simulink model "PAlab3_2_6"  (R2025a)
settings: Solver=VariableStepAuto  StartTime=0.0  StopTime=10.0  RelTol=1e-3
settings Model: Creator=mieszko  LastModifiedBy=Acer

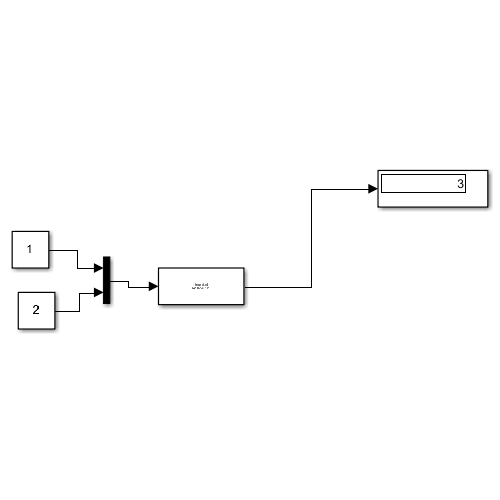
[thumbnail: Simulink's stored preview of the top-level diagram]
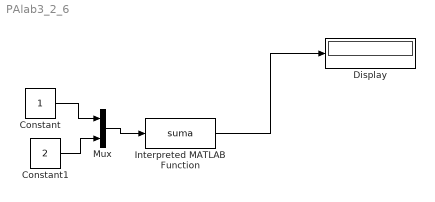
== system PAlab3_2_6 ==
  Constant : Constant
  Constant1 : Constant  Value=2
  Display : Display
  Interpreted MATLAB Function : MATLABFcn  MATLABFcn=suma
  Mux : Mux  Inputs=2
  wires:
  Constant/1 -> Mux/1
  Constant1/1 -> Mux/2
  Mux/1 -> Interpreted MATLAB Function/1
  Interpreted MATLAB Function/1 -> Display/1
